simulink model "example"  (R2015a)
settings: Solver=ode5  SolverMode=SingleTasking  StartTime=0.0  StopTime=600  FixedStep=0.01  RelTol=1e-3  AbsTol=1e-6
undefined symbols (not defined in the file): RTDAC4PCIBaseAddress, T0
libraries: simulink x1
settings Model: SimulationMode=external  ExtModeTrigDuration=50000  ExtModeWriteAllDataToWs=on  Creator=jims  LastModifiedBy=Lab
settings DataIOCC: ExternalInput=[]  InitialState=[]  LimitDataPoints=off  MaxDataPoints=5000  SignalLoggingSaveFormat=ModelDataLogs  SaveOutput=off  SaveTime=off
settings OptimizationCC: BooleanDataType=off  ExpressionDepthLimit=2147483647  InitFltsAndDblsToZero=on
settings DebuggingCC: SaveWithParameterizedLinksMsg=none  UnderspecifiedInitializationDetection=Classic  MergeDetectMultiDrivingBlocksExec=none  SignalResolutionControl=TryResolveAllWithWarning  MultiTaskDSMMsg=warning  MultiTaskCondExecSysMsg=none  IntegerOverflowMsg=none  FcnCallInpInsideContextMsg=UseLocalSettings  StateNameClashWarn=warning  IntegerSaturationMsg=none
settings HardwareCC: ProdBitPerLong=64  ProdBitPerPointer=64  ProdIntDivRoundTo=Zero  ProdEndianess=LittleEndian  ProdWordSize=64  ProdHWDeviceType=Intel->x86-64  TargetBitPerLong=64  TargetBitPerPointer=64  TargetIntDivRoundTo=Zero  TargetEndianess=LittleEndian  TargetWordSize=64  TargetHWDeviceType=Intel->x86-64
settings RTWCC: SystemTargetFile=rtwin.tlc  TemplateMakefile=RTDAC_win.tmf  Description=Real-Time Windows Target
settings RTWinTargetCC: TargetPreCompLibLocation=C:\Program Files\MATLAB\R2015aSP1\toolbox\sldrt\lib\win64  ModelReferenceCompliant=off  CompOptLevelCompliant=off

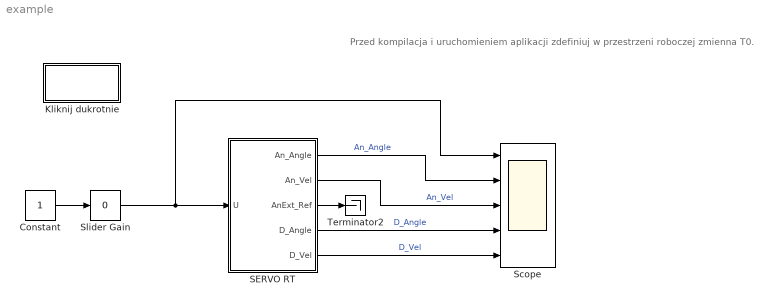
== system example ==
  note: Przed kompilacja i uruchomieniem aplikacji zdefiniuj w przestrzeni roboczej zmienna T0.
  Constant : Constant
  Kliknij dukrotnie : Subsystem
      settings: OpenFcn=T0=0.01
      mask Display: disp('Set T0=0.01')
  SERVO RT : Subsystem
  Scope : Scope  NumInputPorts=5
      settings: TimeRange=15  YMin=-0.493553~-4~0~0~0  YMax=-0.446548~4~130~800~70  SaveName=obiekt  MaxDataPoints=40000  Decimation=2
  Slider Gain : simulink/Math Operations/Slider Gain  low=-1  gain=0  high=1
  Terminator2 : Terminator
  wires:
  SERVO RT/3(AnExt_Ref) -> Terminator2/1
  SERVO RT/1(An_Angle) -> Scope/2  "An_Angle"
  SERVO RT/2(An_Vel) -> Scope/3  "An_Vel"
  SERVO RT/4(D_Angle) -> Scope/4  "D_Angle"
  SERVO RT/5(D_Vel) -> Scope/5  "D_Vel"
  Slider Gain/1 -> SERVO RT/1(U), Scope/1
  Constant/1 -> Slider Gain/1

== system example/Kliknij dukrotnie ==

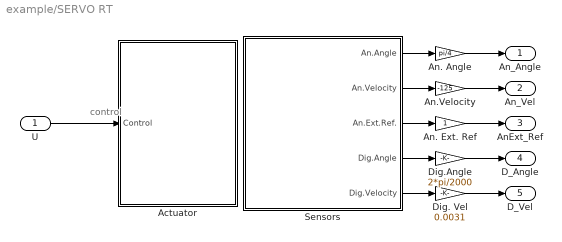
== system example/SERVO RT ==
  note: control
  U : Inport
  Actuator : Subsystem  mask(Servo Input){BaseAddr=RTDAC4PCIBaseAddress, T0=T0}
      mask prompts: BaseAddr "Base Address"; T0 "Sample Time"
      mask help: RTDAC/PCI Device Driver
      mask Display:
      | plot(0,0,55,85,[15,50,50,50,50,50,50,50,50,50,50,50,50,50,15,25,15],[100,100,90,80,75,70,60,50,40,30,25,20,10,0,0,50,100],[15,25],[50,50],[0,0],[20,80]);
      | text(30,47,'ES 151')
      | text(20,7,'RTDAC/PCI')
  An. Angle : Gain  Gain=pi/4  SaturateOnIntegerOverflow=on  OutDataTypeStr=Inherit: Same as input  ParamDataTypeStr=Inherit: Same as input
  An. Ext. Ref : Gain  SaturateOnIntegerOverflow=on  OutDataTypeStr=Inherit: Same as input  ParamDataTypeStr=Inherit: Same as input
  An.Velocity : Gain  Gain=-125  SaturateOnIntegerOverflow=on  OutDataTypeStr=Inherit: Same as input  ParamDataTypeStr=Inherit: Same as input
  Dig. Vel : Gain  Gain=0.0031  SaturateOnIntegerOverflow=on  OutDataTypeStr=Inherit: Same as input  ParamDataTypeStr=Inherit: Same as input
  Dig.Angle : Gain  Gain=2*pi/2000  SaturateOnIntegerOverflow=on  OutDataTypeStr=Inherit: Same as input  ParamDataTypeStr=Inherit: Same as input
  "Sensors                      " : Subsystem  mask(TRMS Output){BaseAddr=RTDAC4PCIBaseAddress, T0=T0}
      mask prompts: BaseAddr "Base address"; T0 "Sample Time"
      mask help: PCL-812 PG Device Driver
      mask Display:
      | plot(0,0,55,85,85-[55,80,80,80,80,80,80,80,80,80,80,80,80,80,55,50,55],[100,100,90,80,75,70,60,50,40,30,25,20,10,0,0,50,100],[55,55],[100,0],[54,55],[50,50]);
      | text(15,47,'ES 151')
      | text(10,7,'RTDAC/PCI')
  An_Angle : Outport
  An_Vel : Outport  Port=2
  AnExt_Ref : Outport  Port=3
  D_Angle : Outport  Port=4
  D_Vel : Outport  Port=5
  wires:
  "Sensors                      "/3(An.Ext.Ref.) -> An. Ext. Ref/1
  "Sensors                      "/1(An.Angle) -> An. Angle/1
  "Sensors                      "/2(An.Velocity) -> An.Velocity/1
  "Sensors                      "/4(Dig.Angle) -> Dig.Angle/1
  "Sensors                      "/5(Dig.Velocity) -> Dig. Vel/1
  Dig.Angle/1 -> D_Angle/1
  U/1 -> Actuator/1(Control)
  An.Velocity/1 -> An_Vel/1
  Dig. Vel/1 -> D_Vel/1
  An. Ext. Ref/1 -> AnExt_Ref/1
  An. Angle/1 -> An_Angle/1

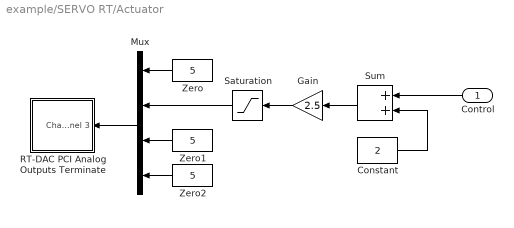
== system example/SERVO RT/Actuator ==
  Control : Inport
  Constant : Constant  Value=2
  Gain : Gain  Gain=2.5  OutDataTypeStr=Inherit: Same as input  ParamDataTypeStr=Inherit: Same as input
  Mux : Mux
  RT-DAC PCI Analog Outputs Terminate : Subsystem  mask(Analog Output Module){BaseAddress=RTDAC4PCIBaseAddress, VoltRange=-10V - +10V, SetOutputsFlag=on, SetOutputsValue=[0 5 0 0], T0=T0}
      mask prompts: BaseAddress "Base Address:"; VoltRange "Voltage Range"; SetOutputsFlag "Set Outputs At Termination"; SetOutputsValue "Termination Outputs [V]:"; T0 "Sample Time (sec):"
      mask help: RT-DAC PCI Device Driver
      mask Help: Set up each field for your specific hardware configuration.
      mask TypeOptions VoltRange: 0V - +10V | -10V - 0V | -10V - +10V
      mask Display: plot(0,0,100,100,[90,80,80,11,11],[90,90,20,20,80],[11,80],[80,80],[80,80],[20,14],[80,85,85,80],[45,45,66,66],[45,45,74,74],[20,13,13,20],[15,27,27,15,15],[75,75,26,26,75],[33,48,48,33,33],[75,75,55,55,75],[55,55,71,71,55],[55,75,75,55,55],[33,41,41,33,33],[50,50,27,27,50],[48,56,56,48,48],[50,50,27,27,50],[62,70,70,62,62],[50,50,27,27,50])
  Saturation : Saturate  UpperLimit=7.5  LowerLimit=2.5
  Sum : Sum  SaturateOnIntegerOverflow=on  InputSameDT=on  OutDataTypeStr=Inherit: Same as first input
  Zero : Constant  Value=5
  Zero1 : Constant  Value=5
  Zero2 : Constant  Value=5
  wires:
  Control/1 -> Sum/1
  Zero/1 -> Mux/1
  Saturation/1 -> Mux/2
  Mux/1 -> RT-DAC PCI Analog Outputs Terminate/1(Channel 0 Channel 1 Channel 2 Channel 3)
  Zero2/1 -> Mux/4
  Zero1/1 -> Mux/3
  Gain/1 -> Saturation/1
  Sum/1 -> Gain/1
  Constant/1 -> Sum/2

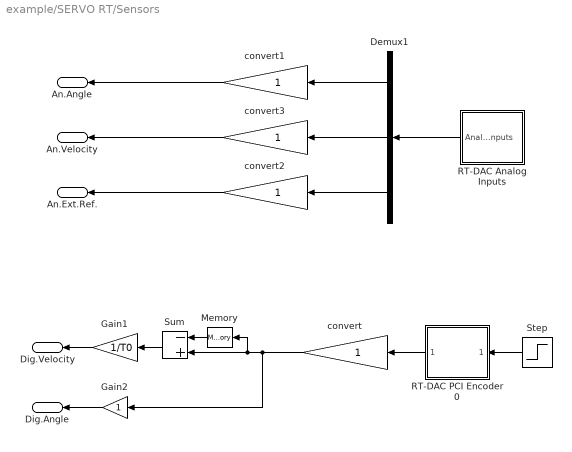
== system example/SERVO RT/Sensors                       ==
  Demux1 : Demux  Outputs=3
  Gain1 : Gain  Gain=1/T0  SaturateOnIntegerOverflow=on  OutDataTypeStr=Inherit: Same as input  ParamDataTypeStr=Inherit: Same as input
  Gain2 : Gain  SaturateOnIntegerOverflow=on  OutDataTypeStr=Inherit: Same as input  ParamDataTypeStr=Inherit: Same as input
  Memory : Memory
  RT-DAC Analog Inputs : Subsystem  mask(Analog Input Module){BaseAddress=RTDAC4PCIBaseAddress, Chan=[10 11 12], Gain=[1 1 1], T0=T0}
      mask prompts: BaseAddress "Base Address:"; Chan "Channel:"; T0 "Sample Time (sec):"
      mask help: RT-DAC PCI Device Driver
      mask Help: Set up each field for your specific hardware configuration.
      mask Display: plot(0,0,100,100,[90,80,80,11,11],[90,90,20,20,80],[11,80],[80,80],[80,80],[20,14],[80,85,85,80],[45,45,66,66],[45,45,74,74],[20,13,13,20],[15,27,27,15,15],[75,75,26,26,75],[33,48,48,33,33],[75,75,55,55,75],[55,55,71,71,55],[55,75,75,55,55],[33,41,41,33,33],[50,50,27,27,50],[48,56,56,48,48],[50,50,27,27,50],[62,70,70,62,62],[50,50,27,27,50])
  "RT-DAC PCI Encoder 0  " : Subsystem  mask(Incremental Encoders){BaseAddress=RTDAC4PCIBaseAddress, ChannelIdx=0, T0=T0}
      mask prompts: BaseAddress "Base Address:"; ChannelIdx "Channel:"; T0 "Sample Time (sec):"
      mask help: RT-DAC PCI Device Driver
      mask Help: Set up each field for your specific hardware configuration.
      mask TypeOptions ChannelIdx: 0 | 1 | 2 | 3
      mask Display: plot(0,0,100,100,[90,80,80,11,11],[90,90,20,20,80],[11,80],[80,80],[80,80],[20,14],[80,85,85,80],[45,45,66,66],[45,45,74,74],[20,13,13,20],[15,27,27,15,15],[75,75,26,26,75],[33,48,48,33,33],[75,75,55,55,75],[55,55,71,71,55],[55,75,75,55,55],[33,41,41,33,33],[50,50,27,27,50],[48,56,56,48,48],[50,50,27,27,50],[62,70,70,62,62],[50,50,27,27,50])
  Step : Step  Time=T0  Before=1  After=0  SampleTime=0
  Sum : Sum  Inputs=-+  SaturateOnIntegerOverflow=on  InputSameDT=on  OutDataTypeStr=Inherit: Same as first input
  convert : Gain  SaturateOnIntegerOverflow=on  OutDataTypeStr=Inherit: Same as input  ParamDataTypeStr=Inherit: Same as input
  convert1 : Gain  SaturateOnIntegerOverflow=on  OutDataTypeStr=Inherit: Same as input  ParamDataTypeStr=Inherit: Same as input
  convert2 : Gain  SaturateOnIntegerOverflow=on  OutDataTypeStr=Inherit: Same as input  ParamDataTypeStr=Inherit: Same as input
  convert3 : Gain  OutDataTypeStr=Inherit: Same as input  ParamDataTypeStr=Inherit: Same as input
  An.Angle : Outport  InitialOutput=0
  An.Velocity : Outport  Port=2  InitialOutput=0
  An.Ext.Ref. : Outport  Port=3  InitialOutput=0
  Dig.Angle : Outport  Port=4  InitialOutput=0
  Dig.Velocity : Outport  Port=5  InitialOutput=0
  wires:
  Gain1/1 -> Dig.Velocity/1
  RT-DAC Analog Inputs/1(Analog Inputs) -> Demux1/1
  Demux1/1 -> convert1/1
  convert1/1 -> An.Angle/1
  Memory/1 -> Sum/1
  convert/1 -> Memory/1, Sum/2, Gain2/1
  Sum/1 -> Gain1/1
  Gain2/1 -> Dig.Angle/1
  Demux1/3 -> convert2/1
  convert2/1 -> An.Ext.Ref./1
  Demux1/2 -> convert3/1
  convert3/1 -> An.Velocity/1
  "RT-DAC PCI Encoder 0  "/1(Encoder Counter) -> convert/1
  Step/1 -> "RT-DAC PCI Encoder 0  "/1(Reset)

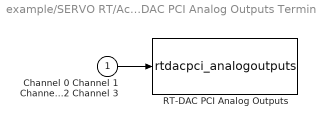
== system example/SERVO RT/Actuator/RT-DAC PCI Analog Outputs Terminate ==
  Channel 0 Channel 1 Channel 2 Channel 3 : Inport
  "RT-DAC PCI Analog Outputs " : S-Function  FunctionName=rtdacpci_analogoutputs  Parameters=BaseAddress, VoltRange, SetOutputsFlag, SetOutputsValue, T0
  wires:
  Channel 0 Channel 1 Channel 2 Channel 3/1 -> "RT-DAC PCI Analog Outputs "/1

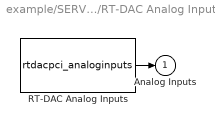
== system example/SERVO RT/Sensors                      /RT-DAC Analog Inputs ==
  RT-DAC Analog Inputs : S-Function  FunctionName=rtdacpci_analoginputs  Parameters=BaseAddress, Chan, Gain, T0
  Analog Inputs : Outport
  wires:
  RT-DAC Analog Inputs/1 -> Analog Inputs/1

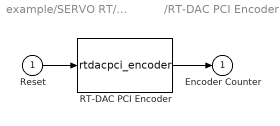
== system example/SERVO RT/Sensors                      /RT-DAC PCI Encoder 0   ==
  Reset : Inport
  RT-DAC PCI Encoder : S-Function  FunctionName=rtdacpci_encoder  Parameters=BaseAddress, ChannelIdx, T0
  Encoder Counter : Outport
  wires:
  RT-DAC PCI Encoder/1 -> Encoder Counter/1
  Reset/1 -> RT-DAC PCI Encoder/1
